simulink model "Mass_Damper_Spring_System"  (R2023a)
settings: Solver=VariableStepAuto  StartTime=0.0  StopTime=20.0  RelTol=1e-3
PreLoadFcn:
  | k = 2;
  | gamma1 = 0.5;
model workspace (MAT data in the model file):
  s = Simulink.Parameter
  s.DataType = 'auto'
  s.Complexity = 'real'
  s.Dimensions = [0 0]
undefined symbols (not defined in the file): beta, gamma2, gamma3, m
settings Model: Creator=geokr  LastModifiedBy=geokr

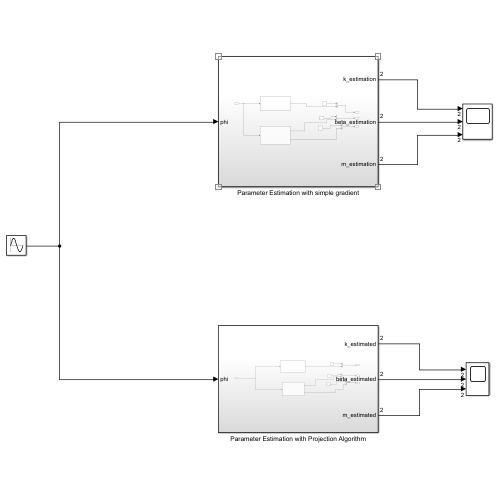
[thumbnail: Simulink's stored preview of the top-level diagram]
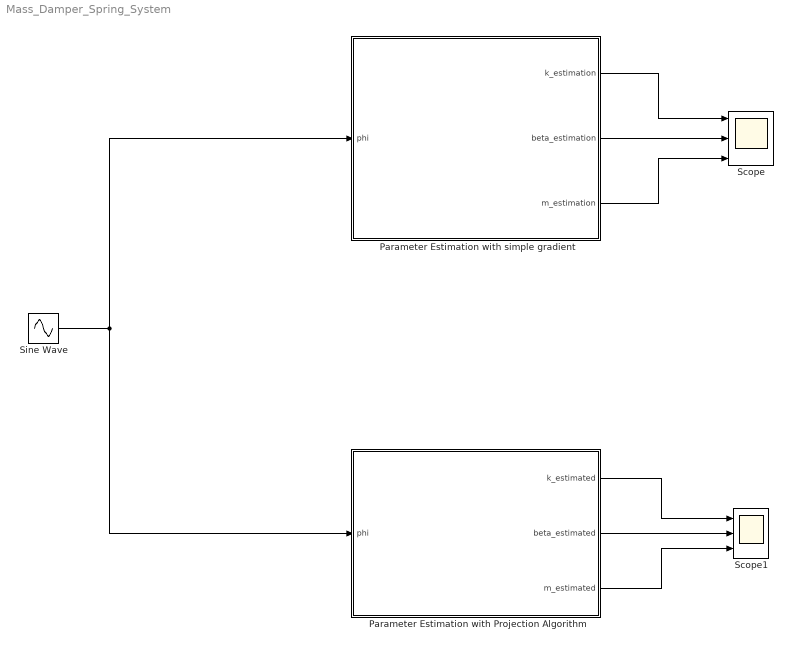
== system Mass_Damper_Spring_System ==
  Parameter Estimation with Projection Algorithm : Subsystem
  Parameter Estimation with simple gradient : Subsystem
  Scope : Scope  NumInputPorts=3
  Scope1 : Scope  NumInputPorts=3
  Sine Wave : Sin  Amplitude=5  Bias=10.5  Frequency=2  SampleTime=0
  wires:
  Sine Wave/1 -> Parameter Estimation with simple gradient/1(phi), Parameter Estimation with Projection Algorithm/1(phi)
  Parameter Estimation with simple gradient/1(k_estimation) -> Scope/1
  Parameter Estimation with simple gradient/2(beta_estimation) -> Scope/2
  Parameter Estimation with simple gradient/3(m_estimation) -> Scope/3
  Parameter Estimation with Projection Algorithm/1(k_estimated) -> Scope1/1
  Parameter Estimation with Projection Algorithm/2(beta_estimated) -> Scope1/2
  Parameter Estimation with Projection Algorithm/3(m_estimated) -> Scope1/3

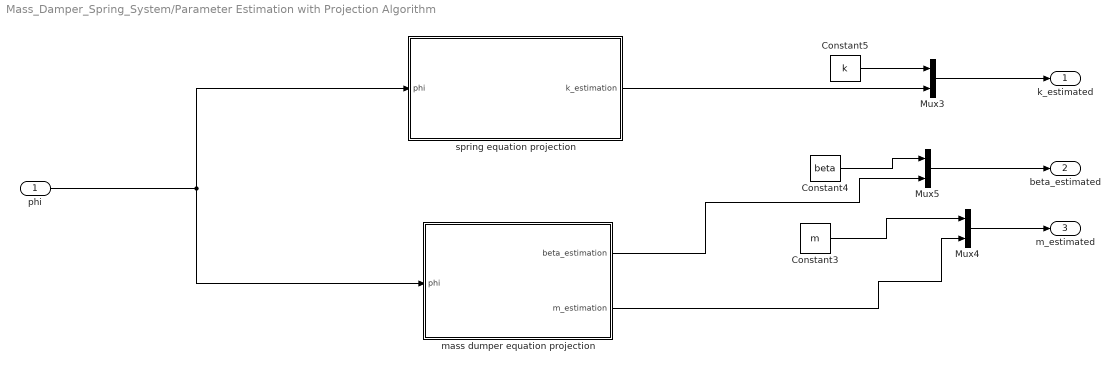
== system Mass_Damper_Spring_System/Parameter Estimation with Projection Algorithm ==
  phi : Inport
  Constant3 : Constant  Value=m
  Constant4 : Constant  Value=beta
  Constant5 : Constant  Value=k
  Mux3 : Mux  Inputs=2
  Mux4 : Mux  Inputs=2
  Mux5 : Mux  Inputs=2
  mass dumper equation projection : Subsystem
  spring equation projection : Subsystem
  k_estimated : Outport
  beta_estimated : Outport  Port=2
  m_estimated : Outport  Port=3
  wires:
  Constant5/1 -> Mux3/1
  Constant3/1 -> Mux4/1
  Constant4/1 -> Mux5/1
  mass dumper equation projection/2(m_estimation) -> Mux4/2
  phi/1 -> spring equation projection/1(phi), mass dumper equation projection/1(phi)
  mass dumper equation projection/1(beta_estimation) -> Mux5/2
  spring equation projection/1(k_estimation) -> Mux3/2
  Mux3/1 -> k_estimated/1
  Mux4/1 -> m_estimated/1
  Mux5/1 -> beta_estimated/1

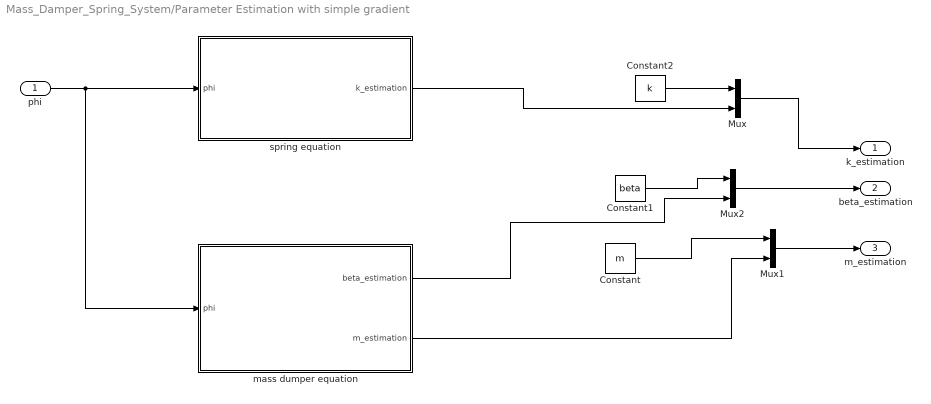
== system Mass_Damper_Spring_System/Parameter Estimation with simple gradient ==
  phi : Inport
  Constant : Constant  Value=m
  Constant1 : Constant  Value=beta
  Constant2 : Constant  Value=k
  Mux : Mux  Inputs=2
  Mux1 : Mux  Inputs=2
  Mux2 : Mux  Inputs=2
  mass dumper equation : Subsystem
  spring equation : Subsystem
  k_estimation : Outport
  beta_estimation : Outport  Port=2
  m_estimation : Outport  Port=3
  wires:
  Constant1/1 -> Mux2/1
  phi/1 -> mass dumper equation/1(phi), spring equation/1(phi)
  Constant2/1 -> Mux/1
  Mux/1 -> k_estimation/1
  Constant/1 -> Mux1/1
  mass dumper equation/2(m_estimation) -> Mux1/2
  Mux1/1 -> m_estimation/1
  mass dumper equation/1(beta_estimation) -> Mux2/2
  spring equation/1(k_estimation) -> Mux/2
  Mux2/1 -> beta_estimation/1

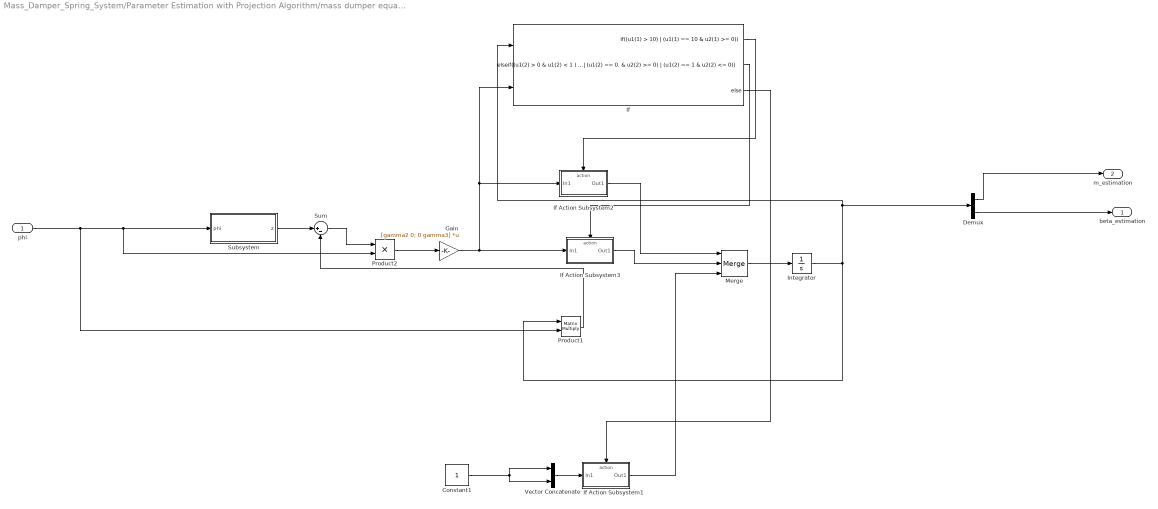
== system Mass_Damper_Spring_System/Parameter Estimation with Projection Algorithm/mass dumper equation projection ==
  phi : Inport
  Constant1 : Constant
  Demux : Demux  Outputs=2
  Gain : Gain  Gain=[gamma2 0; 0 gamma3]  Multiplication=Matrix(K*u)
  If : If  NumInputs=2  IfExpression=(u1(1) > 10) | (u1(1) == 10 & u2(1) >= 0)  ElseIfExpressions=(u1(2) > 0 & u1(2) < 1 ) | (u1(2) == 0. & u2(2) >= 0) | (u1(2) == 1 & u2(2) <= 0)
  If Action Subsystem1 : Subsystem  TreatAsAtomicUnit=on
  If Action Subsystem2 : Subsystem  TreatAsAtomicUnit=on
  If Action Subsystem3 : Subsystem  TreatAsAtomicUnit=on
  Integrator : Integrator
  Merge : Merge  Inputs=3  InitialOutput=1
  Product1 : Product  Multiplication=Matrix(*)
  Product2 : Product
  Subsystem : Subsystem
  Sum : Sum  Inputs=|+-
  Vector Concatenate : Concatenate  Mode=Multidimensional array
  beta_estimation : Outport
  m_estimation : Outport  Port=2
  wires:
  Gain/1 -> If Action Subsystem3/1(In1), If Action Subsystem2/1(In1), If/2
  Integrator/1 -> If/1, Demux/1, Product1/1
  Product1/1 -> Sum/2
  phi/1 -> Subsystem/1(phi), Product2/2, Product1/2
  Product2/1 -> Gain/1
  Sum/1 -> Product2/1
  Demux/1 -> m_estimation/1
  Demux/2 -> beta_estimation/1
  Subsystem/1(z) -> Sum/1
  If/1 -> If Action Subsystem2/Action
  If/3 -> If Action Subsystem1/Action
  Merge/1 -> Integrator/1
  If Action Subsystem1/1(Out1) -> Merge/3
  If Action Subsystem2/1(Out1) -> Merge/1
  Vector Concatenate/1 -> If Action Subsystem1/1(In1)
  Constant1/1 -> Vector Concatenate/2, Vector Concatenate/1
  If/2 -> If Action Subsystem3/Action
  If Action Subsystem3/1(Out1) -> Merge/2

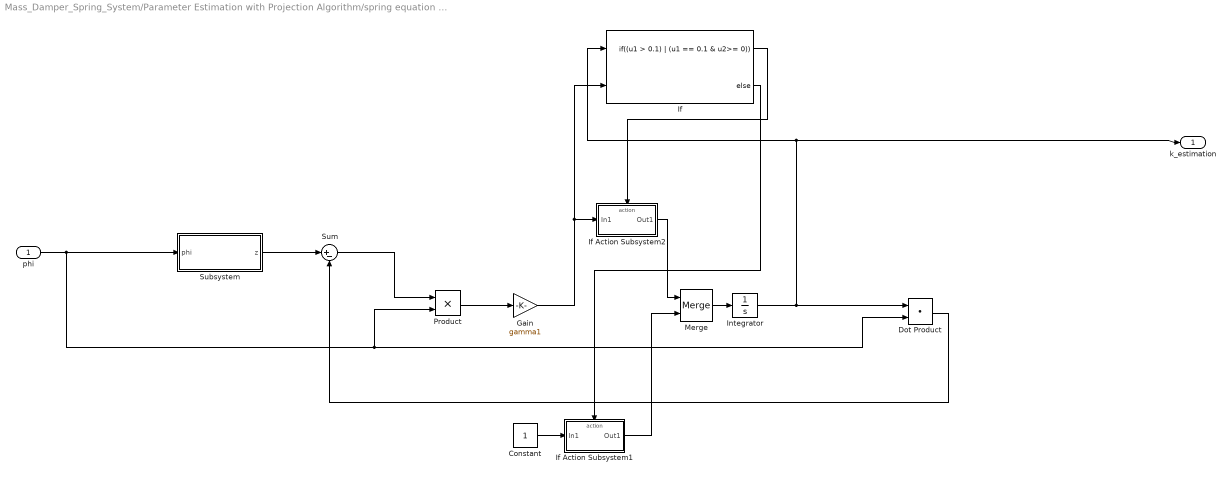
== system Mass_Damper_Spring_System/Parameter Estimation with Projection Algorithm/spring equation projection ==
  phi : Inport
  Constant : Constant
  Dot Product : DotProduct  OutDataTypeStr=Inherit: Inherit via internal rule
  Gain : Gain  Gain=gamma1
  If : If  NumInputs=2  IfExpression=(u1 > 0.1) | (u1 == 0.1 & u2>= 0)
  If Action Subsystem1 : Subsystem  TreatAsAtomicUnit=on
  If Action Subsystem2 : Subsystem  TreatAsAtomicUnit=on
  Integrator : Integrator
  Merge : Merge  InitialOutput=1
  Product : Product
  Subsystem : Subsystem
  Sum : Sum  Inputs=|+-
  k_estimation : Outport
  wires:
  Dot Product/1 -> Sum/2
  Integrator/1 -> If/1, k_estimation/1, Dot Product/1
  Sum/1 -> Product/1
  Product/1 -> Gain/1
  Subsystem/1(z) -> Sum/1
  phi/1 -> Product/2, Dot Product/2, Subsystem/1(phi)
  If/1 -> If Action Subsystem2/Action
  Gain/1 -> If/2, If Action Subsystem2/1(In1)
  Merge/1 -> Integrator/1
  If Action Subsystem2/1(Out1) -> Merge/1
  Constant/1 -> If Action Subsystem1/1(In1)
  If/2 -> If Action Subsystem1/Action
  If Action Subsystem1/1(Out1) -> Merge/2

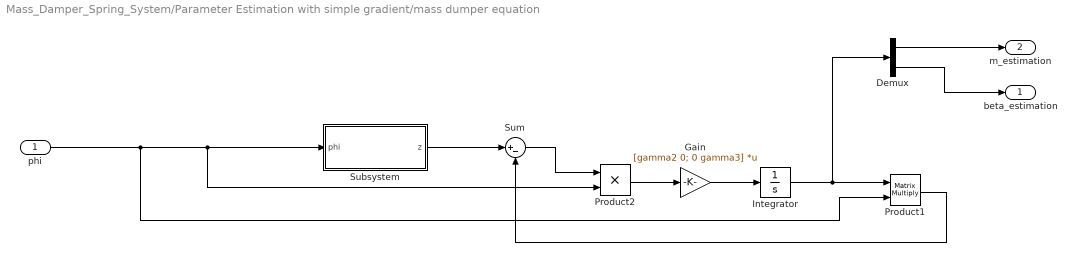
== system Mass_Damper_Spring_System/Parameter Estimation with simple gradient/mass dumper equation ==
  phi : Inport
  Demux : Demux  Outputs=2
  Gain : Gain  Gain=[gamma2 0; 0 gamma3]  Multiplication=Matrix(K*u)
  Integrator : Integrator
  Product1 : Product  Multiplication=Matrix(*)
  Product2 : Product
  Subsystem : Subsystem
  Sum : Sum  Inputs=|+-
  beta_estimation : Outport
  m_estimation : Outport  Port=2
  wires:
  Gain/1 -> Integrator/1
  Integrator/1 -> Demux/1, Product1/1
  Subsystem/1(z) -> Sum/1
  Product1/1 -> Sum/2
  phi/1 -> Product2/2, Subsystem/1(phi), Product1/2
  Product2/1 -> Gain/1
  Sum/1 -> Product2/1
  Demux/1 -> m_estimation/1
  Demux/2 -> beta_estimation/1

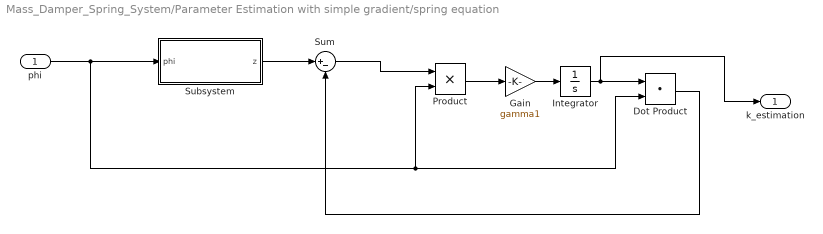
== system Mass_Damper_Spring_System/Parameter Estimation with simple gradient/spring equation ==
  phi : Inport
  Dot Product : DotProduct  OutDataTypeStr=Inherit: Inherit via internal rule
  Gain : Gain  Gain=gamma1
  Integrator : Integrator
  Product : Product
  Subsystem : Subsystem
  Sum : Sum  Inputs=|+-
  k_estimation : Outport
  wires:
  Dot Product/1 -> Sum/2
  Integrator/1 -> k_estimation/1, Dot Product/1
  Sum/1 -> Product/1
  Product/1 -> Gain/1
  Subsystem/1(z) -> Sum/1
  Gain/1 -> Integrator/1
  phi/1 -> Product/2, Dot Product/2, Subsystem/1(phi)

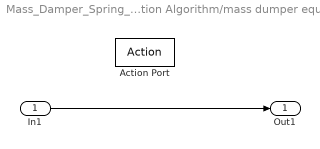
== system Mass_Damper_Spring_System/Parameter Estimation with Projection Algorithm/mass dumper equation projection/If Action Subsystem1 ==
  In1 : Inport
  Action Port : ActionPort  ActionPortLabel=else
  Out1 : Outport
  wires:
  In1/1 -> Out1/1

== system Mass_Damper_Spring_System/Parameter Estimation with Projection Algorithm/mass dumper equation projection/If Action Subsystem2 ==
  In1 : Inport
  Action Port : ActionPort  ActionPortLabel=if((u1(1) > 10) | (u1(1) == 10 & u2(1) >= 0))
  Out1 : Outport
  wires:
  In1/1 -> Out1/1

== system Mass_Damper_Spring_System/Parameter Estimation with Projection Algorithm/mass dumper equation projection/If Action Subsystem3 ==
  In1 : Inport
  Action Port : ActionPort  ActionPortLabel=elseif((u1(2) > 0 & u1(2) < 1 ) | (u1(2) == 0. & u2(2) >= 0) | (u1(2) == 1 & u2(2) <= 0))
  Out1 : Outport
  wires:
  In1/1 -> Out1/1

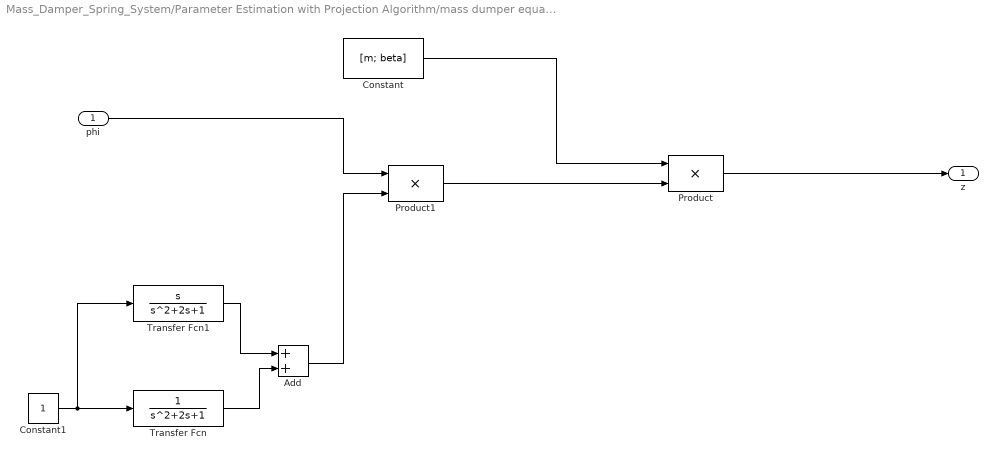
== system Mass_Damper_Spring_System/Parameter Estimation with Projection Algorithm/mass dumper equation projection/Subsystem ==
  phi : Inport
  Add : Sum
  Constant : Constant  Value=[m; beta]  VectorParams1D=off
  Constant1 : Constant
  Product : Product
  Product1 : Product
  Transfer Fcn : TransferFcn  Numerator=[0 0 1]
  Transfer Fcn1 : TransferFcn  Numerator=[0 1 0]
  z : Outport
  wires:
  Product/1 -> z/1
  Constant/1 -> Product/1
  Transfer Fcn1/1 -> Add/1
  Transfer Fcn/1 -> Add/2
  Product1/1 -> Product/2
  phi/1 -> Product1/1
  Constant1/1 -> Transfer Fcn1/1, Transfer Fcn/1
  Add/1 -> Product1/2

== system Mass_Damper_Spring_System/Parameter Estimation with Projection Algorithm/spring equation projection/If Action Subsystem1 ==
  In1 : Inport
  Action Port : ActionPort  ActionPortLabel=else
  Out1 : Outport
  wires:
  In1/1 -> Out1/1

== system Mass_Damper_Spring_System/Parameter Estimation with Projection Algorithm/spring equation projection/If Action Subsystem2 ==
  In1 : Inport
  Action Port : ActionPort  ActionPortLabel=if((u1 > 0.1) | (u1 == 0.1 & u2>= 0))
  Out1 : Outport
  wires:
  In1/1 -> Out1/1

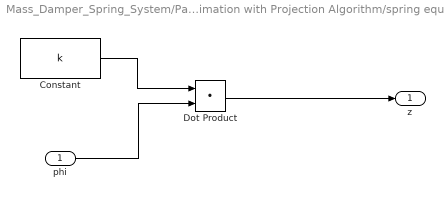
== system Mass_Damper_Spring_System/Parameter Estimation with Projection Algorithm/spring equation projection/Subsystem ==
  phi : Inport
  Constant : Constant  Value=k  VectorParams1D=off
  Dot Product : DotProduct  OutDataTypeStr=Inherit: Inherit via internal rule
  z : Outport
  wires:
  Dot Product/1 -> z/1
  Constant/1 -> Dot Product/1
  phi/1 -> Dot Product/2

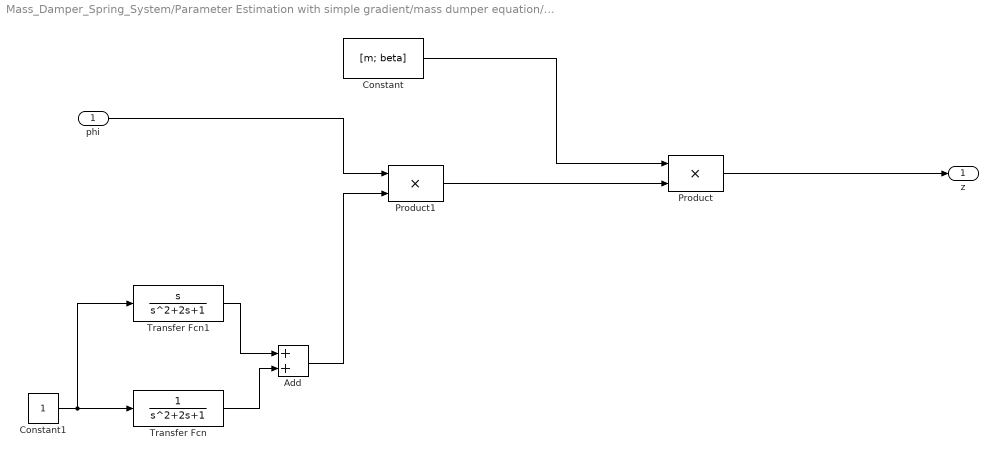
== system Mass_Damper_Spring_System/Parameter Estimation with simple gradient/mass dumper equation/Subsystem ==
  phi : Inport
  Add : Sum
  Constant : Constant  Value=[m; beta]  VectorParams1D=off
  Constant1 : Constant
  Product : Product
  Product1 : Product
  Transfer Fcn : TransferFcn  Numerator=[0 0 1]
  Transfer Fcn1 : TransferFcn  Numerator=[0 1 0]
  z : Outport
  wires:
  Product/1 -> z/1
  Constant/1 -> Product/1
  Transfer Fcn1/1 -> Add/1
  Transfer Fcn/1 -> Add/2
  Product1/1 -> Product/2
  phi/1 -> Product1/1
  Constant1/1 -> Transfer Fcn1/1, Transfer Fcn/1
  Add/1 -> Product1/2

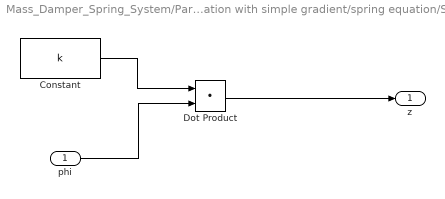
== system Mass_Damper_Spring_System/Parameter Estimation with simple gradient/spring equation/Subsystem ==
  phi : Inport
  Constant : Constant  Value=k  VectorParams1D=off
  Dot Product : DotProduct  OutDataTypeStr=Inherit: Inherit via internal rule
  z : Outport
  wires:
  Dot Product/1 -> z/1
  Constant/1 -> Dot Product/1
  phi/1 -> Dot Product/2
